simulink library "px4_ap1_color_power_led_lib"  (Simulink 9.1)
settings: Solver=VariableStepAuto  StartTime=0.0  StopTime=10.0  RelTol=1e-3
settings Model: Creator=Privat  LastModifiedBy=Privat

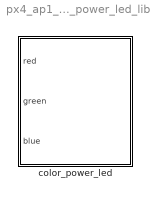
== system px4_ap1_color_power_led_lib ==
  color_power_led : Subsystem  mask(PX4_COLOR_POWER_LED){}
      mask help:
      | Color LED is controlled by three single color channels with value range 0-255. Use simple RGB-Codes for colors.
      | LED Driver use 15 intensity levels for every channel.
      | 0 -15 => off
      | 16-31 => intensity 1
      | 32-47 => intensity 2
      | ...
      mask Display:
      | image(imread('px4_ap1_color_power_led.jpg'));
      | color('red');
      | port_label('input', 1, 'Red');
      | port_label('input', 2, 'Green');
      | port_label('input', 3, 'Blue');

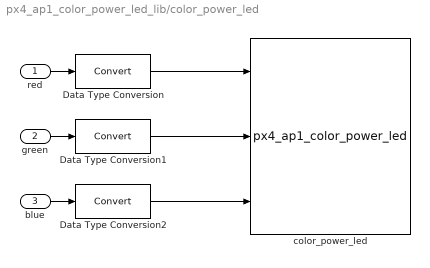
== system px4_ap1_color_power_led_lib/color_power_led ==
  red : Inport
  green : Inport  Port=2
  blue : Inport  Port=3
  Data Type Conversion : DataTypeConversion
  Data Type Conversion1 : DataTypeConversion
  Data Type Conversion2 : DataTypeConversion
  color_power_led : S-Function  FunctionName=px4_ap1_color_power_led  SFunctionDeploymentMode=off  EnableBusSupport=off
  wires:
  Data Type Conversion/1 -> color_power_led/1
  Data Type Conversion1/1 -> color_power_led/2
  Data Type Conversion2/1 -> color_power_led/3
  red/1 -> Data Type Conversion/1
  green/1 -> Data Type Conversion1/1
  blue/1 -> Data Type Conversion2/1
